simulink model "PSB3_0"  (R2021a)
settings: Solver=VariableStepAuto  StartTime=0.0  StopTime=3000  RelTol=1e-3
values from neighbouring files (symbols this model uses):
  n_channel = 1024    [PSB3_0_script.m]    (also in PSB_FPGAdesign8_script.m)
  parallel_factor = 4    [PSB3_0_script.m]    (also in PSB_FPGAdesign8_script.m)
libraries: xbsIndex_r4 x1051, xrbsSSR_Library x154, dspsrcs4 x26
(part 5 of 8)

== system PSB3_0/ov_detector_IFFT_im ==
  rst : Inport
  A : Inport  Port=2
  B : Inport  Port=3
  en : Inport  Port=4
  Constant17 : xbsIndex_r4/Constant  const=1  gui_display_data_type=Boolean  arith_type=Boolean  n_bits=16  bin_pt=14  preci_type=Single  exp_width=8  frac_width=24  explicit_period=on  period=1  equ=P=C  opselect=C  inp2=PCIN>>17  opr=+  inp1=P  carry=CIN  dbl_ovrd=off  block_type=constant
  Demux : Demux  Outputs=8
  Expression : xbsIndex_r4/Expression  expression=a1 | b1 | c1 | d1 | a2 | b2 | c2 | d2  align_bp=off  en=off  latency=1  precision=Full  arith_type=Unsigned  n_bits=1  bin_pt=0  dbl_ovrd=off  block_type=expr
  Register : xbsIndex_r4/Register  init=0  rst=on  en=on  dbl_ovrd=off  block_type=register
  Vector Absolute : xrbsSSR_Library/vector Absolute  precision=User Defined  arith_type="Signed  (2's comp)"  n_bits=20  bin_pt=15  quantization=Truncate  overflow=Saturate  en=off  sg_latency=1  dbl_ovrd=off  block_type=abs_ssr  sg_ssr_name=vect_absolute  sg_ssr=8  sg_ssr_prev=8
      settings: SourceProductName=Xilinx SSR Blockset
  Vector Absolute1 : xrbsSSR_Library/vector Absolute  precision=User Defined  arith_type="Signed  (2's comp)"  n_bits=20  bin_pt=15  quantization=Truncate  overflow=Saturate  en=off  sg_latency=1  dbl_ovrd=off  block_type=abs_ssr  sg_ssr_name=vect_absolute  sg_ssr=8  sg_ssr_prev=8
      settings: SourceProductName=Xilinx SSR Blockset
  Vector Register : xrbsSSR_Library/Vector Register  init=zeros(1,8)  en=on  rst=on  sg_ssr=8  sg_ssr_prev=8  sg_ssr_name=vect_reg  block_type=register_ssr  dbl_ovrd=off
      settings: SourceProductName=Xilinx SSR Blockset
  Vector Relational : xrbsSSR_Library/Vector Relational  mode=a>b  op_type=Bool  en=off  sg_latency=1  dbl_ovrd=off  has_advanced_contorl=0  block_type=relational_ssr  sg_ssr=8  sg_ssr_prev=8  sg_ssr_name=vect_relational
      settings: SourceProductName=Xilinx SSR Blockset
  ov : Outport
  wires:
  Demux/8 -> Expression/8
  Demux/7 -> Expression/7
  Demux/6 -> Expression/6
  Demux/5 -> Expression/5
  Demux/4 -> Expression/4
  Demux/3 -> Expression/3
  B/1 -> Vector Absolute1/1
  Vector Absolute1/1 -> Vector Relational/2
  Vector Absolute/1 -> Vector Relational/1
  Vector Register/1 -> Vector Absolute/1
  en/1 -> Vector Register/3
  A/1 -> Vector Register/1
  rst/1 -> Register/2, Vector Register/2
  Demux/1 -> Expression/1
  Vector Relational/1 -> Demux/1
  Register/1 -> ov/1
  Demux/2 -> Expression/2
  Constant17/1 -> Register/1
  Expression/1 -> Register/3

== system PSB3_0/ov_detector_IFFT_re ==
  rst : Inport
  A : Inport  Port=2
  B : Inport  Port=3
  en : Inport  Port=4
  Constant17 : xbsIndex_r4/Constant  const=1  gui_display_data_type=Boolean  arith_type=Boolean  n_bits=16  bin_pt=14  preci_type=Single  exp_width=8  frac_width=24  explicit_period=on  period=1  equ=P=C  opselect=C  inp2=PCIN>>17  opr=+  inp1=P  carry=CIN  dbl_ovrd=off  block_type=constant
  Demux : Demux  Outputs=8
  Expression : xbsIndex_r4/Expression  expression=a1 | b1 | c1 | d1 | a2 | b2 | c2 | d2  align_bp=off  en=off  latency=1  precision=Full  arith_type=Unsigned  n_bits=1  bin_pt=0  dbl_ovrd=off  block_type=expr
  Register : xbsIndex_r4/Register  init=0  rst=on  en=on  dbl_ovrd=off  block_type=register
  Vector Absolute : xrbsSSR_Library/vector Absolute  precision=User Defined  arith_type="Signed  (2's comp)"  n_bits=20  bin_pt=15  quantization=Truncate  overflow=Saturate  en=off  sg_latency=1  dbl_ovrd=off  block_type=abs_ssr  sg_ssr_name=vect_absolute  sg_ssr=8  sg_ssr_prev=8
      settings: SourceProductName=Xilinx SSR Blockset
  Vector Absolute1 : xrbsSSR_Library/vector Absolute  precision=User Defined  arith_type="Signed  (2's comp)"  n_bits=20  bin_pt=15  quantization=Truncate  overflow=Saturate  en=off  sg_latency=1  dbl_ovrd=off  block_type=abs_ssr  sg_ssr_name=vect_absolute  sg_ssr=8  sg_ssr_prev=8
      settings: SourceProductName=Xilinx SSR Blockset
  Vector Register : xrbsSSR_Library/Vector Register  init=zeros(1,8)  en=on  rst=on  sg_ssr=8  sg_ssr_prev=8  sg_ssr_name=vect_reg  block_type=register_ssr  dbl_ovrd=off
      settings: SourceProductName=Xilinx SSR Blockset
  Vector Relational : xrbsSSR_Library/Vector Relational  mode=a>b  op_type=Bool  en=off  sg_latency=1  dbl_ovrd=off  has_advanced_contorl=0  block_type=relational_ssr  sg_ssr=8  sg_ssr_prev=8  sg_ssr_name=vect_relational
      settings: SourceProductName=Xilinx SSR Blockset
  ov : Outport
  wires:
  Expression/1 -> Register/3
  Constant17/1 -> Register/1
  Demux/2 -> Expression/2
  Register/1 -> ov/1
  Vector Relational/1 -> Demux/1
  Demux/1 -> Expression/1
  rst/1 -> Vector Register/2, Register/2
  A/1 -> Vector Register/1
  en/1 -> Vector Register/3
  Vector Register/1 -> Vector Absolute/1
  Vector Absolute/1 -> Vector Relational/1
  Vector Absolute1/1 -> Vector Relational/2
  B/1 -> Vector Absolute1/1
  Demux/3 -> Expression/3
  Demux/4 -> Expression/4
  Demux/5 -> Expression/5
  Demux/6 -> Expression/6
  Demux/7 -> Expression/7
  Demux/8 -> Expression/8

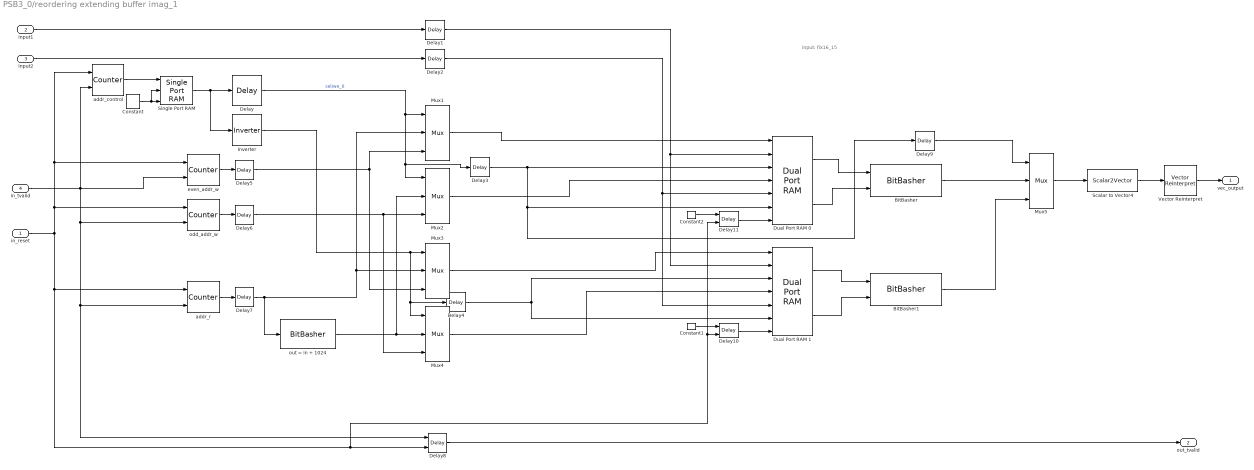
== system PSB3_0/reordering extending buffer imag_1 ==
  note: input: fix16_15
  in_reset : Inport
  input1 : Inport  Port=2
  input2 : Inport  Port=3
  in_tvalid : Inport  Port=4
  BitBasher : xbsIndex_r4/BitBasher  bitexpr=out = {8{b,a}}  display_expr=on  sr_1=out  arith_type1=Unsigned  bin_pt1=0  sr_2=2  arith_type2=Unsigned  bin_pt2=0  sr_3=3  arith_type3=Unsigned  bin_pt3=0  sr_4=4  arith_type4=Unsigned  bin_pt4=0  dbl_ovrd=off  block_type=bitbasher
  BitBasher1 : xbsIndex_r4/BitBasher  bitexpr=out = {8{b,a}}  display_expr=on  sr_1=out  arith_type1=Unsigned  bin_pt1=0  sr_2=2  arith_type2=Unsigned  bin_pt2=0  sr_3=3  arith_type3=Unsigned  bin_pt3=0  sr_4=4  arith_type4=Unsigned  bin_pt4=0  dbl_ovrd=off  block_type=bitbasher
  Constant : xbsIndex_r4/Constant  const=0  gui_display_data_type=Boolean  arith_type=Boolean  n_bits=16  bin_pt=14  preci_type=Single  exp_width=8  frac_width=24  explicit_period=on  period=1  equ=P=C  opselect=C  inp2=PCIN>>17  opr=+  inp1=P  carry=CIN  dbl_ovrd=off  block_type=constant
  Constant1 : xbsIndex_r4/Constant  const=1  gui_display_data_type=Boolean  arith_type=Boolean  n_bits=16  bin_pt=14  preci_type=Single  exp_width=8  frac_width=24  explicit_period=on  period=1  equ=P=C  opselect=C  inp2=PCIN>>17  opr=+  inp1=P  carry=CIN  dbl_ovrd=off  block_type=constant
  Constant2 : xbsIndex_r4/Constant  const=1  gui_display_data_type=Boolean  arith_type=Boolean  n_bits=16  bin_pt=14  preci_type=Single  exp_width=8  frac_width=24  explicit_period=on  period=1  equ=P=C  opselect=C  inp2=PCIN>>17  opr=+  inp1=P  carry=CIN  dbl_ovrd=off  block_type=constant
  Delay{,3..4,9} (4 alike) : xbsIndex_r4/Delay  rst=off  infoeditControl=Selection of Reset will increase slice count due to use of real FFs and instead of SRLs  en=off  latency=1  reg_retiming=off  dbl_ovrd=off  block_type=delay
  Delay1 : xbsIndex_r4/Delay  rst=off  infoeditControl=Selection of Reset will increase slice count due to use of real FFs and instead of SRLs  en=off  latency=3  reg_retiming=off  dbl_ovrd=off  block_type=delay
  Delay10 : xbsIndex_r4/Delay  rst=on  infoeditControl=Selection of Reset will increase slice count due to use of real FFs and instead of SRLs  en=off  latency=1000  reg_retiming=off  dbl_ovrd=off  block_type=delay
  Delay11 : xbsIndex_r4/Delay  rst=on  infoeditControl=Selection of Reset will increase slice count due to use of real FFs and instead of SRLs  en=off  latency=1000  reg_retiming=off  dbl_ovrd=off  block_type=delay
  Delay2 : xbsIndex_r4/Delay  rst=off  infoeditControl=Selection of Reset will increase slice count due to use of real FFs and instead of SRLs  en=off  latency=3  reg_retiming=off  dbl_ovrd=off  block_type=delay
  Delay5 : xbsIndex_r4/Delay  rst=off  infoeditControl=Selection of Reset will increase slice count due to use of real FFs and instead of SRLs  en=off  latency=2  reg_retiming=off  dbl_ovrd=off  block_type=delay
  Delay6 : xbsIndex_r4/Delay  rst=off  infoeditControl=Selection of Reset will increase slice count due to use of real FFs and instead of SRLs  en=off  latency=2  reg_retiming=off  dbl_ovrd=off  block_type=delay
  Delay7 : xbsIndex_r4/Delay  rst=off  infoeditControl=Selection of Reset will increase slice count due to use of real FFs and instead of SRLs  en=off  latency=2  reg_retiming=off  dbl_ovrd=off  block_type=delay
  Delay8 : xbsIndex_r4/Delay  rst=on  infoeditControl=Selection of Reset will increase slice count due to use of real FFs and instead of SRLs  en=off  latency=4+1024/parallel_factor+1 - 2  reg_retiming=off  dbl_ovrd=off  block_type=delay
  Dual Port RAM 0 : xbsIndex_r4/Dual Port RAM  depth=2048/parallel_factor  initVector=1  distributed_mem=Block RAM  init_a=0  init_b=0  rst_a=off  rst_b=off  en_a=off  en_b=on  latency=1  write_mode_A=Read Before Write  write_mode_B=Read Before Write  optimize=Area  dbl_ovrd=off  simulation_type=fast_sim  block_type=dpram
  Dual Port RAM 1 : xbsIndex_r4/Dual Port RAM  depth=2048/parallel_factor  initVector=1  distributed_mem=Block RAM  init_a=0  init_b=0  rst_a=off  rst_b=off  en_a=off  en_b=on  latency=1  write_mode_A=Read Before Write  write_mode_B=Read Before Write  optimize=Area  dbl_ovrd=off  simulation_type=fast_sim  block_type=dpram
  Inverter : xbsIndex_r4/Inverter  en=off  latency=1  dbl_ovrd=off  block_type=inv
  Mux{1..4} (4 alike) : xbsIndex_r4/Mux  inputs=2  en=off  latency=1  precision=Full  arith_type=Unsigned  n_bits=16  bin_pt=14  quantization=Truncate  overflow=Wrap  dbl_ovrd=off  block_type=mux
  Mux5 : xbsIndex_r4/Mux  inputs=2  en=off  latency=1  precision=User Defined  arith_type=Unsigned  n_bits=256  bin_pt=0  quantization=Truncate  overflow=Flag as error  dbl_ovrd=off  block_type=mux
  Scalar to Vector4 : xrbsSSR_Library/Scalar2Vector  Width=16  sg_ssr=16  sg_ssr_prev=16  sg_ssr_name=vect_Scalar2Vector  block_type=scalar2vector_ssr
      settings: SourceProductName=Xilinx SSR Blockset
  Single Port RAM : xbsIndex_r4/Single Port RAM  depth=2048/parallel_factor  initVector=[ones(1,1024/parallel_factor), zeros(1,1024/parallel_factor)]  distributed_mem=Block RAM  write_mode=Read Before Write  rst=off  init_reg=0  en=off  optimize_latency=off  latency=1  optimize=Area  dbl_ovrd=off  simulation_type=fast_sim  block_type=spram
  Vector Reinterpret : xrbsSSR_Library/Vector Reinterpret  sg_ssr=16  sg_ssr_prev=16  force_arith_type=on  arith_type="Signed  (2's comp)"  force_bin_pt=on  bin_pt=15  block_type=reinterpret_ssr
      settings: SourceProductName=Xilinx SSR Blockset  infoedit="The Vector Reinterpret block Changes vector input signal type without altering the binary representation. You can change the signal between signed and unsigned, and relocate the binary point.<br><br>Hardware notes: In hardware this block costs nothing.<br><br>Example:  Suppose the input is 6 bits wide, signed, with 2 fractional bits, and the output is forced to unsigned with 0 fractional bits.  Then an input of -2.0 (1110.00 in binary 2's complement) becomes an output of 56 (111000 in binary)."
  addr_control : xbsIndex_r4/Counter  cnt_type=Free Running  cnt_to=Inf  operation=Up  start_count=0  cnt_by_val=1  arith_type=Unsigned  n_bits=11-2  bin_pt=0  load_pin=off  rst=on  en=on  explicit_period=on  period=1  use_behavioral_HDL=off  implementation=Fabric  dbl_ovrd=off  block_type=counter
  addr_r : xbsIndex_r4/Counter  cnt_type=Free Running  cnt_to=Inf  operation=Up  start_count=0  cnt_by_val=1  arith_type=Unsigned  n_bits=10-2  bin_pt=0  load_pin=off  rst=on  en=on  explicit_period=on  period=1  use_behavioral_HDL=off  implementation=Fabric  dbl_ovrd=off  block_type=counter
  even_addr_w : xbsIndex_r4/Counter  cnt_type=Free Running  cnt_to=Inf  operation=Up  start_count=0  cnt_by_val=2  arith_type=Unsigned  n_bits=11-2  bin_pt=0  load_pin=off  rst=on  en=on  explicit_period=on  period=1  use_behavioral_HDL=off  implementation=Fabric  dbl_ovrd=off  block_type=counter
  odd_addr_w : xbsIndex_r4/Counter  cnt_type=Free Running  cnt_to=Inf  operation=Up  start_count=1  cnt_by_val=2  arith_type=Unsigned  n_bits=11-2  bin_pt=0  load_pin=off  rst=on  en=on  explicit_period=on  period=1  use_behavioral_HDL=off  implementation=Fabric  dbl_ovrd=off  block_type=counter
  out = in + 1024 : xbsIndex_r4/BitBasher  bitexpr=out={1'b1, in}  display_expr=on  sr_1=out  arith_type1=Unsigned  bin_pt1=0  sr_2=2  arith_type2=Unsigned  bin_pt2=0  sr_3=3  arith_type3=Unsigned  bin_pt3=0  sr_4=4  arith_type4=Unsigned  bin_pt4=0  dbl_ovrd=off  block_type=bitbasher
  vec_output : Outport
  out_tvalid : Outport  Port=2
  wires:
  in_reset/1 -> addr_control/1, even_addr_w/1, odd_addr_w/1, addr_r/1, Delay8/2, Delay10/2, Delay11/2
  Vector Reinterpret/1 -> vec_output/1
  Dual Port RAM 1/2 -> BitBasher1/2
  Dual Port RAM 0/2 -> BitBasher/2
  Delay10/1 -> Dual Port RAM 1/7
  Constant1/1 -> Delay10/1
  Delay11/1 -> Dual Port RAM 0/7
  Constant2/1 -> Delay11/1
  input2/1 -> Delay2/1
  input1/1 -> Delay1/1
  Scalar to Vector4/1 -> Vector Reinterpret/1
  BitBasher1/1 -> Mux5/3
  Delay4/1 -> Dual Port RAM 1/3, Dual Port RAM 1/6
  BitBasher/1 -> Mux5/2
  Delay5/1 -> Mux1/3, Mux3/3
  addr_control/1 -> Single Port RAM/1
  Delay2/1 -> Dual Port RAM 0/5, Dual Port RAM 1/5
  out = in + 1024/1 -> Mux4/2, Mux2/2
  Constant/1 -> Single Port RAM/3, Single Port RAM/2
  Inverter/1 -> Mux3/1, Mux4/1, Delay4/1
  Delay3/1 -> Delay9/1, Dual Port RAM 0/6, Dual Port RAM 0/3
  Single Port RAM/1 -> Delay/1, Inverter/1
  Mux3/1 -> Dual Port RAM 1/1
  Dual Port RAM 1/1 -> BitBasher1/1
  addr_r/1 -> Delay7/1
  Delay7/1 -> out = in + 1024/1, Mux3/2, Mux1/2
  Mux1/1 -> Dual Port RAM 0/1
  Mux5/1 -> Scalar to Vector4/1
  even_addr_w/1 -> Delay5/1
  Delay/1 -> Mux1/1, Mux2/1, Delay3/1  "sel/we_0"
  Delay8/1 -> out_tvalid/1
  Delay9/1 -> Mux5/1
  odd_addr_w/1 -> Delay6/1
  Mux4/1 -> Dual Port RAM 1/4
  in_tvalid/1 -> addr_control/2, even_addr_w/2, odd_addr_w/2, Delay8/1, addr_r/2
  Mux2/1 -> Dual Port RAM 0/4
  Delay1/1 -> Dual Port RAM 0/2, Dual Port RAM 1/2
  Dual Port RAM 0/1 -> BitBasher/1
  Delay6/1 -> Mux2/3, Mux4/3

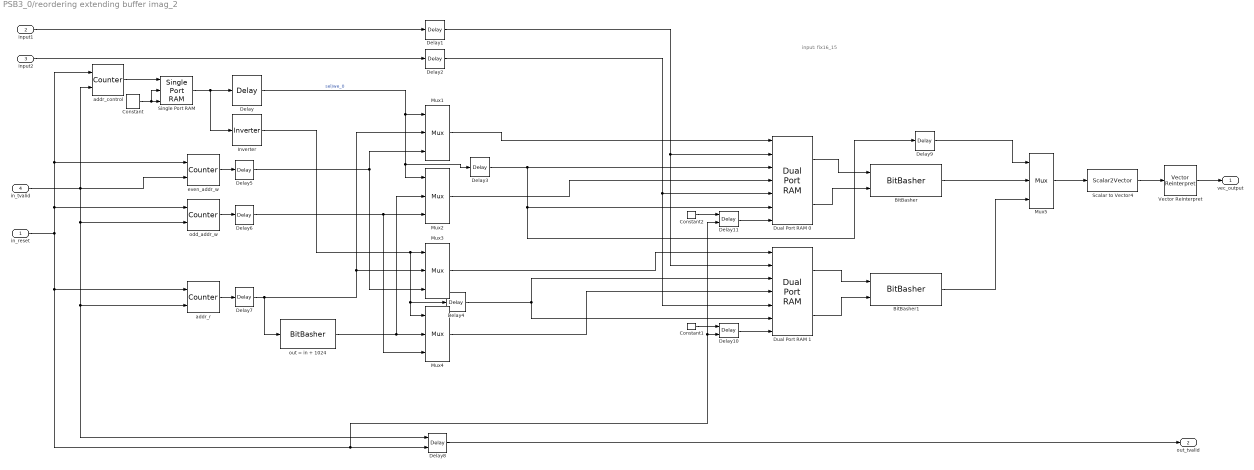
== system PSB3_0/reordering extending buffer imag_2 ==
  note: input: fix16_15
  in_reset : Inport
  input1 : Inport  Port=2
  input2 : Inport  Port=3
  in_tvalid : Inport  Port=4
  BitBasher : xbsIndex_r4/BitBasher  bitexpr=out = {8{b,a}}  display_expr=on  sr_1=out  arith_type1=Unsigned  bin_pt1=0  sr_2=2  arith_type2=Unsigned  bin_pt2=0  sr_3=3  arith_type3=Unsigned  bin_pt3=0  sr_4=4  arith_type4=Unsigned  bin_pt4=0  dbl_ovrd=off  block_type=bitbasher
  BitBasher1 : xbsIndex_r4/BitBasher  bitexpr=out = {8{b,a}}  display_expr=on  sr_1=out  arith_type1=Unsigned  bin_pt1=0  sr_2=2  arith_type2=Unsigned  bin_pt2=0  sr_3=3  arith_type3=Unsigned  bin_pt3=0  sr_4=4  arith_type4=Unsigned  bin_pt4=0  dbl_ovrd=off  block_type=bitbasher
  Constant : xbsIndex_r4/Constant  const=0  gui_display_data_type=Boolean  arith_type=Boolean  n_bits=16  bin_pt=14  preci_type=Single  exp_width=8  frac_width=24  explicit_period=on  period=1  equ=P=C  opselect=C  inp2=PCIN>>17  opr=+  inp1=P  carry=CIN  dbl_ovrd=off  block_type=constant
  Constant1 : xbsIndex_r4/Constant  const=1  gui_display_data_type=Boolean  arith_type=Boolean  n_bits=16  bin_pt=14  preci_type=Single  exp_width=8  frac_width=24  explicit_period=on  period=1  equ=P=C  opselect=C  inp2=PCIN>>17  opr=+  inp1=P  carry=CIN  dbl_ovrd=off  block_type=constant
  Constant2 : xbsIndex_r4/Constant  const=1  gui_display_data_type=Boolean  arith_type=Boolean  n_bits=16  bin_pt=14  preci_type=Single  exp_width=8  frac_width=24  explicit_period=on  period=1  equ=P=C  opselect=C  inp2=PCIN>>17  opr=+  inp1=P  carry=CIN  dbl_ovrd=off  block_type=constant
  Delay{,3..4,9} (4 alike) : xbsIndex_r4/Delay  rst=off  infoeditControl=Selection of Reset will increase slice count due to use of real FFs and instead of SRLs  en=off  latency=1  reg_retiming=off  dbl_ovrd=off  block_type=delay
  Delay1 : xbsIndex_r4/Delay  rst=off  infoeditControl=Selection of Reset will increase slice count due to use of real FFs and instead of SRLs  en=off  latency=3  reg_retiming=off  dbl_ovrd=off  block_type=delay
  Delay10 : xbsIndex_r4/Delay  rst=on  infoeditControl=Selection of Reset will increase slice count due to use of real FFs and instead of SRLs  en=off  latency=1000  reg_retiming=off  dbl_ovrd=off  block_type=delay
  Delay11 : xbsIndex_r4/Delay  rst=on  infoeditControl=Selection of Reset will increase slice count due to use of real FFs and instead of SRLs  en=off  latency=1000  reg_retiming=off  dbl_ovrd=off  block_type=delay
  Delay2 : xbsIndex_r4/Delay  rst=off  infoeditControl=Selection of Reset will increase slice count due to use of real FFs and instead of SRLs  en=off  latency=3  reg_retiming=off  dbl_ovrd=off  block_type=delay
  Delay5 : xbsIndex_r4/Delay  rst=off  infoeditControl=Selection of Reset will increase slice count due to use of real FFs and instead of SRLs  en=off  latency=2  reg_retiming=off  dbl_ovrd=off  block_type=delay
  Delay6 : xbsIndex_r4/Delay  rst=off  infoeditControl=Selection of Reset will increase slice count due to use of real FFs and instead of SRLs  en=off  latency=2  reg_retiming=off  dbl_ovrd=off  block_type=delay
  Delay7 : xbsIndex_r4/Delay  rst=off  infoeditControl=Selection of Reset will increase slice count due to use of real FFs and instead of SRLs  en=off  latency=2  reg_retiming=off  dbl_ovrd=off  block_type=delay
  Delay8 : xbsIndex_r4/Delay  rst=on  infoeditControl=Selection of Reset will increase slice count due to use of real FFs and instead of SRLs  en=off  latency=4+1024/parallel_factor+1 - 2  reg_retiming=off  dbl_ovrd=off  block_type=delay
  Dual Port RAM 0 : xbsIndex_r4/Dual Port RAM  depth=2048/parallel_factor  initVector=1  distributed_mem=Block RAM  init_a=0  init_b=0  rst_a=off  rst_b=off  en_a=off  en_b=on  latency=1  write_mode_A=Read Before Write  write_mode_B=Read Before Write  optimize=Area  dbl_ovrd=off  simulation_type=fast_sim  block_type=dpram
  Dual Port RAM 1 : xbsIndex_r4/Dual Port RAM  depth=2048/parallel_factor  initVector=1  distributed_mem=Block RAM  init_a=0  init_b=0  rst_a=off  rst_b=off  en_a=off  en_b=on  latency=1  write_mode_A=Read Before Write  write_mode_B=Read Before Write  optimize=Area  dbl_ovrd=off  simulation_type=fast_sim  block_type=dpram
  Inverter : xbsIndex_r4/Inverter  en=off  latency=1  dbl_ovrd=off  block_type=inv
  Mux{1..4} (4 alike) : xbsIndex_r4/Mux  inputs=2  en=off  latency=1  precision=Full  arith_type=Unsigned  n_bits=16  bin_pt=14  quantization=Truncate  overflow=Wrap  dbl_ovrd=off  block_type=mux
  Mux5 : xbsIndex_r4/Mux  inputs=2  en=off  latency=1  precision=User Defined  arith_type=Unsigned  n_bits=256  bin_pt=0  quantization=Truncate  overflow=Flag as error  dbl_ovrd=off  block_type=mux
  Scalar to Vector4 : xrbsSSR_Library/Scalar2Vector  Width=16  sg_ssr=16  sg_ssr_prev=16  sg_ssr_name=vect_Scalar2Vector  block_type=scalar2vector_ssr
      settings: SourceProductName=Xilinx SSR Blockset
  Single Port RAM : xbsIndex_r4/Single Port RAM  depth=2048/parallel_factor  initVector=[ones(1,1024/parallel_factor), zeros(1,1024/parallel_factor)]  distributed_mem=Block RAM  write_mode=Read Before Write  rst=off  init_reg=0  en=off  optimize_latency=off  latency=1  optimize=Area  dbl_ovrd=off  simulation_type=fast_sim  block_type=spram
  Vector Reinterpret : xrbsSSR_Library/Vector Reinterpret  sg_ssr=16  sg_ssr_prev=16  force_arith_type=on  arith_type="Signed  (2's comp)"  force_bin_pt=on  bin_pt=15  block_type=reinterpret_ssr
      settings: SourceProductName=Xilinx SSR Blockset  infoedit="The Vector Reinterpret block Changes vector input signal type without altering the binary representation. You can change the signal between signed and unsigned, and relocate the binary point.<br><br>Hardware notes: In hardware this block costs nothing.<br><br>Example:  Suppose the input is 6 bits wide, signed, with 2 fractional bits, and the output is forced to unsigned with 0 fractional bits.  Then an input of -2.0 (1110.00 in binary 2's complement) becomes an output of 56 (111000 in binary)."
  addr_control : xbsIndex_r4/Counter  cnt_type=Free Running  cnt_to=Inf  operation=Up  start_count=0  cnt_by_val=1  arith_type=Unsigned  n_bits=11-2  bin_pt=0  load_pin=off  rst=on  en=on  explicit_period=on  period=1  use_behavioral_HDL=off  implementation=Fabric  dbl_ovrd=off  block_type=counter
  addr_r : xbsIndex_r4/Counter  cnt_type=Free Running  cnt_to=Inf  operation=Up  start_count=0  cnt_by_val=1  arith_type=Unsigned  n_bits=10-2  bin_pt=0  load_pin=off  rst=on  en=on  explicit_period=on  period=1  use_behavioral_HDL=off  implementation=Fabric  dbl_ovrd=off  block_type=counter
  even_addr_w : xbsIndex_r4/Counter  cnt_type=Free Running  cnt_to=Inf  operation=Up  start_count=0  cnt_by_val=2  arith_type=Unsigned  n_bits=11-2  bin_pt=0  load_pin=off  rst=on  en=on  explicit_period=on  period=1  use_behavioral_HDL=off  implementation=Fabric  dbl_ovrd=off  block_type=counter
  odd_addr_w : xbsIndex_r4/Counter  cnt_type=Free Running  cnt_to=Inf  operation=Up  start_count=1  cnt_by_val=2  arith_type=Unsigned  n_bits=11-2  bin_pt=0  load_pin=off  rst=on  en=on  explicit_period=on  period=1  use_behavioral_HDL=off  implementation=Fabric  dbl_ovrd=off  block_type=counter
  out = in + 1024 : xbsIndex_r4/BitBasher  bitexpr=out={1'b1, in}  display_expr=on  sr_1=out  arith_type1=Unsigned  bin_pt1=0  sr_2=2  arith_type2=Unsigned  bin_pt2=0  sr_3=3  arith_type3=Unsigned  bin_pt3=0  sr_4=4  arith_type4=Unsigned  bin_pt4=0  dbl_ovrd=off  block_type=bitbasher
  vec_output : Outport
  out_tvalid : Outport  Port=2
  wires:
  in_reset/1 -> addr_control/1, even_addr_w/1, odd_addr_w/1, addr_r/1, Delay8/2, Delay10/2, Delay11/2
  Vector Reinterpret/1 -> vec_output/1
  Dual Port RAM 1/2 -> BitBasher1/2
  Dual Port RAM 0/2 -> BitBasher/2
  Delay10/1 -> Dual Port RAM 1/7
  Constant1/1 -> Delay10/1
  Delay11/1 -> Dual Port RAM 0/7
  Constant2/1 -> Delay11/1
  input2/1 -> Delay2/1
  input1/1 -> Delay1/1
  Scalar to Vector4/1 -> Vector Reinterpret/1
  BitBasher1/1 -> Mux5/3
  Delay4/1 -> Dual Port RAM 1/3, Dual Port RAM 1/6
  BitBasher/1 -> Mux5/2
  Delay5/1 -> Mux1/3, Mux3/3
  addr_control/1 -> Single Port RAM/1
  Delay2/1 -> Dual Port RAM 0/5, Dual Port RAM 1/5
  out = in + 1024/1 -> Mux4/2, Mux2/2
  Constant/1 -> Single Port RAM/3, Single Port RAM/2
  Inverter/1 -> Mux3/1, Mux4/1, Delay4/1
  Delay3/1 -> Delay9/1, Dual Port RAM 0/6, Dual Port RAM 0/3
  Single Port RAM/1 -> Delay/1, Inverter/1
  Mux3/1 -> Dual Port RAM 1/1
  Dual Port RAM 1/1 -> BitBasher1/1
  addr_r/1 -> Delay7/1
  Delay7/1 -> out = in + 1024/1, Mux3/2, Mux1/2
  Mux1/1 -> Dual Port RAM 0/1
  Mux5/1 -> Scalar to Vector4/1
  even_addr_w/1 -> Delay5/1
  Delay/1 -> Mux1/1, Mux2/1, Delay3/1  "sel/we_0"
  Delay8/1 -> out_tvalid/1
  Delay9/1 -> Mux5/1
  odd_addr_w/1 -> Delay6/1
  Mux4/1 -> Dual Port RAM 1/4
  in_tvalid/1 -> addr_control/2, even_addr_w/2, odd_addr_w/2, Delay8/1, addr_r/2
  Mux2/1 -> Dual Port RAM 0/4
  Delay1/1 -> Dual Port RAM 0/2, Dual Port RAM 1/2
  Dual Port RAM 0/1 -> BitBasher/1
  Delay6/1 -> Mux2/3, Mux4/3

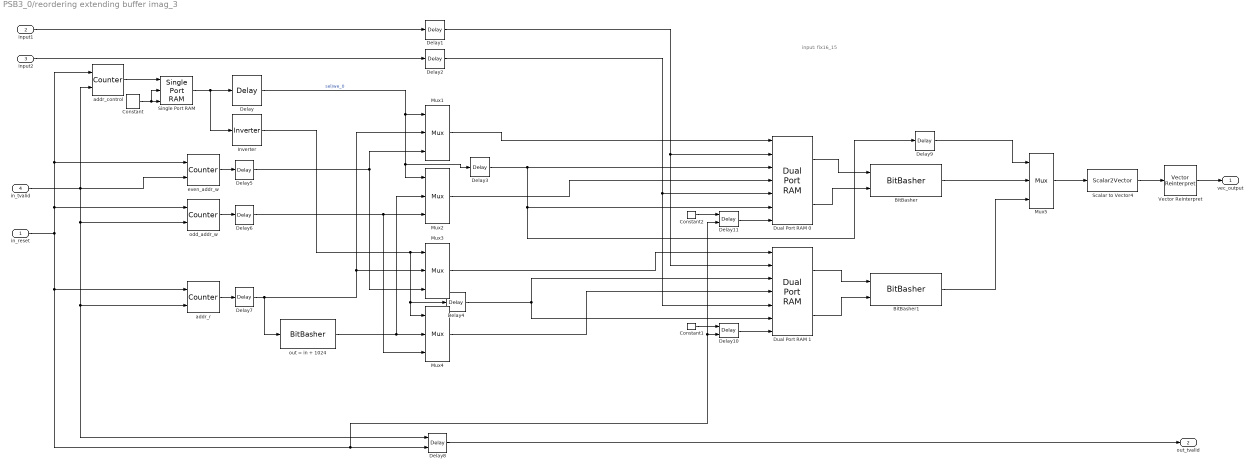
== system PSB3_0/reordering extending buffer imag_3 ==
  note: input: fix16_15
  in_reset : Inport
  input1 : Inport  Port=2
  input2 : Inport  Port=3
  in_tvalid : Inport  Port=4
  BitBasher : xbsIndex_r4/BitBasher  bitexpr=out = {8{b,a}}  display_expr=on  sr_1=out  arith_type1=Unsigned  bin_pt1=0  sr_2=2  arith_type2=Unsigned  bin_pt2=0  sr_3=3  arith_type3=Unsigned  bin_pt3=0  sr_4=4  arith_type4=Unsigned  bin_pt4=0  dbl_ovrd=off  block_type=bitbasher
  BitBasher1 : xbsIndex_r4/BitBasher  bitexpr=out = {8{b,a}}  display_expr=on  sr_1=out  arith_type1=Unsigned  bin_pt1=0  sr_2=2  arith_type2=Unsigned  bin_pt2=0  sr_3=3  arith_type3=Unsigned  bin_pt3=0  sr_4=4  arith_type4=Unsigned  bin_pt4=0  dbl_ovrd=off  block_type=bitbasher
  Constant : xbsIndex_r4/Constant  const=0  gui_display_data_type=Boolean  arith_type=Boolean  n_bits=16  bin_pt=14  preci_type=Single  exp_width=8  frac_width=24  explicit_period=on  period=1  equ=P=C  opselect=C  inp2=PCIN>>17  opr=+  inp1=P  carry=CIN  dbl_ovrd=off  block_type=constant
  Constant1 : xbsIndex_r4/Constant  const=1  gui_display_data_type=Boolean  arith_type=Boolean  n_bits=16  bin_pt=14  preci_type=Single  exp_width=8  frac_width=24  explicit_period=on  period=1  equ=P=C  opselect=C  inp2=PCIN>>17  opr=+  inp1=P  carry=CIN  dbl_ovrd=off  block_type=constant
  Constant2 : xbsIndex_r4/Constant  const=1  gui_display_data_type=Boolean  arith_type=Boolean  n_bits=16  bin_pt=14  preci_type=Single  exp_width=8  frac_width=24  explicit_period=on  period=1  equ=P=C  opselect=C  inp2=PCIN>>17  opr=+  inp1=P  carry=CIN  dbl_ovrd=off  block_type=constant
  Delay{,3..4,9} (4 alike) : xbsIndex_r4/Delay  rst=off  infoeditControl=Selection of Reset will increase slice count due to use of real FFs and instead of SRLs  en=off  latency=1  reg_retiming=off  dbl_ovrd=off  block_type=delay
  Delay1 : xbsIndex_r4/Delay  rst=off  infoeditControl=Selection of Reset will increase slice count due to use of real FFs and instead of SRLs  en=off  latency=3  reg_retiming=off  dbl_ovrd=off  block_type=delay
  Delay10 : xbsIndex_r4/Delay  rst=on  infoeditControl=Selection of Reset will increase slice count due to use of real FFs and instead of SRLs  en=off  latency=1000  reg_retiming=off  dbl_ovrd=off  block_type=delay
  Delay11 : xbsIndex_r4/Delay  rst=on  infoeditControl=Selection of Reset will increase slice count due to use of real FFs and instead of SRLs  en=off  latency=1000  reg_retiming=off  dbl_ovrd=off  block_type=delay
  Delay2 : xbsIndex_r4/Delay  rst=off  infoeditControl=Selection of Reset will increase slice count due to use of real FFs and instead of SRLs  en=off  latency=3  reg_retiming=off  dbl_ovrd=off  block_type=delay
  Delay5 : xbsIndex_r4/Delay  rst=off  infoeditControl=Selection of Reset will increase slice count due to use of real FFs and instead of SRLs  en=off  latency=2  reg_retiming=off  dbl_ovrd=off  block_type=delay
  Delay6 : xbsIndex_r4/Delay  rst=off  infoeditControl=Selection of Reset will increase slice count due to use of real FFs and instead of SRLs  en=off  latency=2  reg_retiming=off  dbl_ovrd=off  block_type=delay
  Delay7 : xbsIndex_r4/Delay  rst=off  infoeditControl=Selection of Reset will increase slice count due to use of real FFs and instead of SRLs  en=off  latency=2  reg_retiming=off  dbl_ovrd=off  block_type=delay
  Delay8 : xbsIndex_r4/Delay  rst=on  infoeditControl=Selection of Reset will increase slice count due to use of real FFs and instead of SRLs  en=off  latency=4+1024/parallel_factor+1 - 2  reg_retiming=off  dbl_ovrd=off  block_type=delay
  Dual Port RAM 0 : xbsIndex_r4/Dual Port RAM  depth=2048/parallel_factor  initVector=1  distributed_mem=Block RAM  init_a=0  init_b=0  rst_a=off  rst_b=off  en_a=off  en_b=on  latency=1  write_mode_A=Read Before Write  write_mode_B=Read Before Write  optimize=Area  dbl_ovrd=off  simulation_type=fast_sim  block_type=dpram
  Dual Port RAM 1 : xbsIndex_r4/Dual Port RAM  depth=2048/parallel_factor  initVector=1  distributed_mem=Block RAM  init_a=0  init_b=0  rst_a=off  rst_b=off  en_a=off  en_b=on  latency=1  write_mode_A=Read Before Write  write_mode_B=Read Before Write  optimize=Area  dbl_ovrd=off  simulation_type=fast_sim  block_type=dpram
  Inverter : xbsIndex_r4/Inverter  en=off  latency=1  dbl_ovrd=off  block_type=inv
  Mux{1..4} (4 alike) : xbsIndex_r4/Mux  inputs=2  en=off  latency=1  precision=Full  arith_type=Unsigned  n_bits=16  bin_pt=14  quantization=Truncate  overflow=Wrap  dbl_ovrd=off  block_type=mux
  Mux5 : xbsIndex_r4/Mux  inputs=2  en=off  latency=1  precision=User Defined  arith_type=Unsigned  n_bits=256  bin_pt=0  quantization=Truncate  overflow=Flag as error  dbl_ovrd=off  block_type=mux
  Scalar to Vector4 : xrbsSSR_Library/Scalar2Vector  Width=16  sg_ssr=16  sg_ssr_prev=16  sg_ssr_name=vect_Scalar2Vector  block_type=scalar2vector_ssr
      settings: SourceProductName=Xilinx SSR Blockset
  Single Port RAM : xbsIndex_r4/Single Port RAM  depth=2048/parallel_factor  initVector=[ones(1,1024/parallel_factor), zeros(1,1024/parallel_factor)]  distributed_mem=Block RAM  write_mode=Read Before Write  rst=off  init_reg=0  en=off  optimize_latency=off  latency=1  optimize=Area  dbl_ovrd=off  simulation_type=fast_sim  block_type=spram
  Vector Reinterpret : xrbsSSR_Library/Vector Reinterpret  sg_ssr=16  sg_ssr_prev=16  force_arith_type=on  arith_type="Signed  (2's comp)"  force_bin_pt=on  bin_pt=15  block_type=reinterpret_ssr
      settings: SourceProductName=Xilinx SSR Blockset  infoedit="The Vector Reinterpret block Changes vector input signal type without altering the binary representation. You can change the signal between signed and unsigned, and relocate the binary point.<br><br>Hardware notes: In hardware this block costs nothing.<br><br>Example:  Suppose the input is 6 bits wide, signed, with 2 fractional bits, and the output is forced to unsigned with 0 fractional bits.  Then an input of -2.0 (1110.00 in binary 2's complement) becomes an output of 56 (111000 in binary)."
  addr_control : xbsIndex_r4/Counter  cnt_type=Free Running  cnt_to=Inf  operation=Up  start_count=0  cnt_by_val=1  arith_type=Unsigned  n_bits=11-2  bin_pt=0  load_pin=off  rst=on  en=on  explicit_period=on  period=1  use_behavioral_HDL=off  implementation=Fabric  dbl_ovrd=off  block_type=counter
  addr_r : xbsIndex_r4/Counter  cnt_type=Free Running  cnt_to=Inf  operation=Up  start_count=0  cnt_by_val=1  arith_type=Unsigned  n_bits=10-2  bin_pt=0  load_pin=off  rst=on  en=on  explicit_period=on  period=1  use_behavioral_HDL=off  implementation=Fabric  dbl_ovrd=off  block_type=counter
  even_addr_w : xbsIndex_r4/Counter  cnt_type=Free Running  cnt_to=Inf  operation=Up  start_count=0  cnt_by_val=2  arith_type=Unsigned  n_bits=11-2  bin_pt=0  load_pin=off  rst=on  en=on  explicit_period=on  period=1  use_behavioral_HDL=off  implementation=Fabric  dbl_ovrd=off  block_type=counter
  odd_addr_w : xbsIndex_r4/Counter  cnt_type=Free Running  cnt_to=Inf  operation=Up  start_count=1  cnt_by_val=2  arith_type=Unsigned  n_bits=11-2  bin_pt=0  load_pin=off  rst=on  en=on  explicit_period=on  period=1  use_behavioral_HDL=off  implementation=Fabric  dbl_ovrd=off  block_type=counter
  out = in + 1024 : xbsIndex_r4/BitBasher  bitexpr=out={1'b1, in}  display_expr=on  sr_1=out  arith_type1=Unsigned  bin_pt1=0  sr_2=2  arith_type2=Unsigned  bin_pt2=0  sr_3=3  arith_type3=Unsigned  bin_pt3=0  sr_4=4  arith_type4=Unsigned  bin_pt4=0  dbl_ovrd=off  block_type=bitbasher
  vec_output : Outport
  out_tvalid : Outport  Port=2
  wires:
  in_reset/1 -> addr_control/1, even_addr_w/1, odd_addr_w/1, addr_r/1, Delay8/2, Delay10/2, Delay11/2
  Vector Reinterpret/1 -> vec_output/1
  Dual Port RAM 1/2 -> BitBasher1/2
  Dual Port RAM 0/2 -> BitBasher/2
  Delay10/1 -> Dual Port RAM 1/7
  Constant1/1 -> Delay10/1
  Delay11/1 -> Dual Port RAM 0/7
  Constant2/1 -> Delay11/1
  input2/1 -> Delay2/1
  input1/1 -> Delay1/1
  Scalar to Vector4/1 -> Vector Reinterpret/1
  BitBasher1/1 -> Mux5/3
  Delay4/1 -> Dual Port RAM 1/3, Dual Port RAM 1/6
  BitBasher/1 -> Mux5/2
  Delay5/1 -> Mux1/3, Mux3/3
  addr_control/1 -> Single Port RAM/1
  Delay2/1 -> Dual Port RAM 0/5, Dual Port RAM 1/5
  out = in + 1024/1 -> Mux4/2, Mux2/2
  Constant/1 -> Single Port RAM/3, Single Port RAM/2
  Inverter/1 -> Mux3/1, Mux4/1, Delay4/1
  Delay3/1 -> Delay9/1, Dual Port RAM 0/6, Dual Port RAM 0/3
  Single Port RAM/1 -> Delay/1, Inverter/1
  Mux3/1 -> Dual Port RAM 1/1
  Dual Port RAM 1/1 -> BitBasher1/1
  addr_r/1 -> Delay7/1
  Delay7/1 -> out = in + 1024/1, Mux3/2, Mux1/2
  Mux1/1 -> Dual Port RAM 0/1
  Mux5/1 -> Scalar to Vector4/1
  even_addr_w/1 -> Delay5/1
  Delay/1 -> Mux1/1, Mux2/1, Delay3/1  "sel/we_0"
  Delay8/1 -> out_tvalid/1
  Delay9/1 -> Mux5/1
  odd_addr_w/1 -> Delay6/1
  Mux4/1 -> Dual Port RAM 1/4
  in_tvalid/1 -> addr_control/2, even_addr_w/2, odd_addr_w/2, Delay8/1, addr_r/2
  Mux2/1 -> Dual Port RAM 0/4
  Delay1/1 -> Dual Port RAM 0/2, Dual Port RAM 1/2
  Dual Port RAM 0/1 -> BitBasher/1
  Delay6/1 -> Mux2/3, Mux4/3

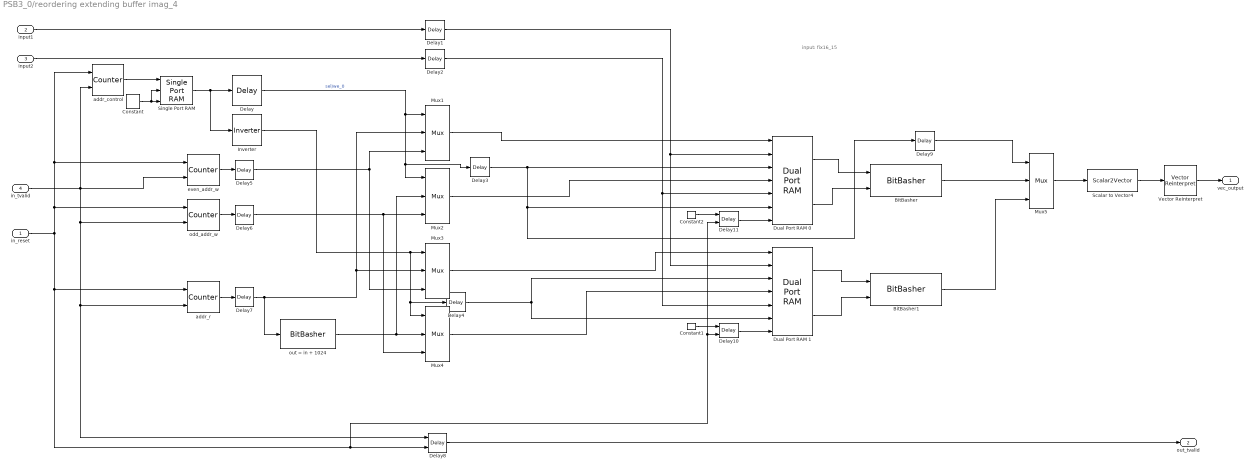
== system PSB3_0/reordering extending buffer imag_4 ==
  note: input: fix16_15
  in_reset : Inport
  input1 : Inport  Port=2
  input2 : Inport  Port=3
  in_tvalid : Inport  Port=4
  BitBasher : xbsIndex_r4/BitBasher  bitexpr=out = {8{b,a}}  display_expr=on  sr_1=out  arith_type1=Unsigned  bin_pt1=0  sr_2=2  arith_type2=Unsigned  bin_pt2=0  sr_3=3  arith_type3=Unsigned  bin_pt3=0  sr_4=4  arith_type4=Unsigned  bin_pt4=0  dbl_ovrd=off  block_type=bitbasher
  BitBasher1 : xbsIndex_r4/BitBasher  bitexpr=out = {8{b,a}}  display_expr=on  sr_1=out  arith_type1=Unsigned  bin_pt1=0  sr_2=2  arith_type2=Unsigned  bin_pt2=0  sr_3=3  arith_type3=Unsigned  bin_pt3=0  sr_4=4  arith_type4=Unsigned  bin_pt4=0  dbl_ovrd=off  block_type=bitbasher
  Constant : xbsIndex_r4/Constant  const=0  gui_display_data_type=Boolean  arith_type=Boolean  n_bits=16  bin_pt=14  preci_type=Single  exp_width=8  frac_width=24  explicit_period=on  period=1  equ=P=C  opselect=C  inp2=PCIN>>17  opr=+  inp1=P  carry=CIN  dbl_ovrd=off  block_type=constant
  Constant1 : xbsIndex_r4/Constant  const=1  gui_display_data_type=Boolean  arith_type=Boolean  n_bits=16  bin_pt=14  preci_type=Single  exp_width=8  frac_width=24  explicit_period=on  period=1  equ=P=C  opselect=C  inp2=PCIN>>17  opr=+  inp1=P  carry=CIN  dbl_ovrd=off  block_type=constant
  Constant2 : xbsIndex_r4/Constant  const=1  gui_display_data_type=Boolean  arith_type=Boolean  n_bits=16  bin_pt=14  preci_type=Single  exp_width=8  frac_width=24  explicit_period=on  period=1  equ=P=C  opselect=C  inp2=PCIN>>17  opr=+  inp1=P  carry=CIN  dbl_ovrd=off  block_type=constant
  Delay{,3..4,9} (4 alike) : xbsIndex_r4/Delay  rst=off  infoeditControl=Selection of Reset will increase slice count due to use of real FFs and instead of SRLs  en=off  latency=1  reg_retiming=off  dbl_ovrd=off  block_type=delay
  Delay1 : xbsIndex_r4/Delay  rst=off  infoeditControl=Selection of Reset will increase slice count due to use of real FFs and instead of SRLs  en=off  latency=3  reg_retiming=off  dbl_ovrd=off  block_type=delay
  Delay10 : xbsIndex_r4/Delay  rst=on  infoeditControl=Selection of Reset will increase slice count due to use of real FFs and instead of SRLs  en=off  latency=1000  reg_retiming=off  dbl_ovrd=off  block_type=delay
  Delay11 : xbsIndex_r4/Delay  rst=on  infoeditControl=Selection of Reset will increase slice count due to use of real FFs and instead of SRLs  en=off  latency=1000  reg_retiming=off  dbl_ovrd=off  block_type=delay
  Delay2 : xbsIndex_r4/Delay  rst=off  infoeditControl=Selection of Reset will increase slice count due to use of real FFs and instead of SRLs  en=off  latency=3  reg_retiming=off  dbl_ovrd=off  block_type=delay
  Delay5 : xbsIndex_r4/Delay  rst=off  infoeditControl=Selection of Reset will increase slice count due to use of real FFs and instead of SRLs  en=off  latency=2  reg_retiming=off  dbl_ovrd=off  block_type=delay
  Delay6 : xbsIndex_r4/Delay  rst=off  infoeditControl=Selection of Reset will increase slice count due to use of real FFs and instead of SRLs  en=off  latency=2  reg_retiming=off  dbl_ovrd=off  block_type=delay
  Delay7 : xbsIndex_r4/Delay  rst=off  infoeditControl=Selection of Reset will increase slice count due to use of real FFs and instead of SRLs  en=off  latency=2  reg_retiming=off  dbl_ovrd=off  block_type=delay
  Delay8 : xbsIndex_r4/Delay  rst=on  infoeditControl=Selection of Reset will increase slice count due to use of real FFs and instead of SRLs  en=off  latency=4+1024/parallel_factor+1 - 2  reg_retiming=off  dbl_ovrd=off  block_type=delay
  Dual Port RAM 0 : xbsIndex_r4/Dual Port RAM  depth=2048/parallel_factor  initVector=1  distributed_mem=Block RAM  init_a=0  init_b=0  rst_a=off  rst_b=off  en_a=off  en_b=on  latency=1  write_mode_A=Read Before Write  write_mode_B=Read Before Write  optimize=Area  dbl_ovrd=off  simulation_type=fast_sim  block_type=dpram
  Dual Port RAM 1 : xbsIndex_r4/Dual Port RAM  depth=2048/parallel_factor  initVector=1  distributed_mem=Block RAM  init_a=0  init_b=0  rst_a=off  rst_b=off  en_a=off  en_b=on  latency=1  write_mode_A=Read Before Write  write_mode_B=Read Before Write  optimize=Area  dbl_ovrd=off  simulation_type=fast_sim  block_type=dpram
  Inverter : xbsIndex_r4/Inverter  en=off  latency=1  dbl_ovrd=off  block_type=inv
  Mux{1..4} (4 alike) : xbsIndex_r4/Mux  inputs=2  en=off  latency=1  precision=Full  arith_type=Unsigned  n_bits=16  bin_pt=14  quantization=Truncate  overflow=Wrap  dbl_ovrd=off  block_type=mux
  Mux5 : xbsIndex_r4/Mux  inputs=2  en=off  latency=1  precision=User Defined  arith_type=Unsigned  n_bits=256  bin_pt=0  quantization=Truncate  overflow=Flag as error  dbl_ovrd=off  block_type=mux
  Scalar to Vector4 : xrbsSSR_Library/Scalar2Vector  Width=16  sg_ssr=16  sg_ssr_prev=16  sg_ssr_name=vect_Scalar2Vector  block_type=scalar2vector_ssr
      settings: SourceProductName=Xilinx SSR Blockset
  Single Port RAM : xbsIndex_r4/Single Port RAM  depth=2048/parallel_factor  initVector=[ones(1,1024/parallel_factor), zeros(1,1024/parallel_factor)]  distributed_mem=Block RAM  write_mode=Read Before Write  rst=off  init_reg=0  en=off  optimize_latency=off  latency=1  optimize=Area  dbl_ovrd=off  simulation_type=fast_sim  block_type=spram
  Vector Reinterpret : xrbsSSR_Library/Vector Reinterpret  sg_ssr=16  sg_ssr_prev=16  force_arith_type=on  arith_type="Signed  (2's comp)"  force_bin_pt=on  bin_pt=15  block_type=reinterpret_ssr
      settings: SourceProductName=Xilinx SSR Blockset  infoedit="The Vector Reinterpret block Changes vector input signal type without altering the binary representation. You can change the signal between signed and unsigned, and relocate the binary point.<br><br>Hardware notes: In hardware this block costs nothing.<br><br>Example:  Suppose the input is 6 bits wide, signed, with 2 fractional bits, and the output is forced to unsigned with 0 fractional bits.  Then an input of -2.0 (1110.00 in binary 2's complement) becomes an output of 56 (111000 in binary)."
  addr_control : xbsIndex_r4/Counter  cnt_type=Free Running  cnt_to=Inf  operation=Up  start_count=0  cnt_by_val=1  arith_type=Unsigned  n_bits=11-2  bin_pt=0  load_pin=off  rst=on  en=on  explicit_period=on  period=1  use_behavioral_HDL=off  implementation=Fabric  dbl_ovrd=off  block_type=counter
  addr_r : xbsIndex_r4/Counter  cnt_type=Free Running  cnt_to=Inf  operation=Up  start_count=0  cnt_by_val=1  arith_type=Unsigned  n_bits=10-2  bin_pt=0  load_pin=off  rst=on  en=on  explicit_period=on  period=1  use_behavioral_HDL=off  implementation=Fabric  dbl_ovrd=off  block_type=counter
  even_addr_w : xbsIndex_r4/Counter  cnt_type=Free Running  cnt_to=Inf  operation=Up  start_count=0  cnt_by_val=2  arith_type=Unsigned  n_bits=11-2  bin_pt=0  load_pin=off  rst=on  en=on  explicit_period=on  period=1  use_behavioral_HDL=off  implementation=Fabric  dbl_ovrd=off  block_type=counter
  odd_addr_w : xbsIndex_r4/Counter  cnt_type=Free Running  cnt_to=Inf  operation=Up  start_count=1  cnt_by_val=2  arith_type=Unsigned  n_bits=11-2  bin_pt=0  load_pin=off  rst=on  en=on  explicit_period=on  period=1  use_behavioral_HDL=off  implementation=Fabric  dbl_ovrd=off  block_type=counter
  out = in + 1024 : xbsIndex_r4/BitBasher  bitexpr=out={1'b1, in}  display_expr=on  sr_1=out  arith_type1=Unsigned  bin_pt1=0  sr_2=2  arith_type2=Unsigned  bin_pt2=0  sr_3=3  arith_type3=Unsigned  bin_pt3=0  sr_4=4  arith_type4=Unsigned  bin_pt4=0  dbl_ovrd=off  block_type=bitbasher
  vec_output : Outport
  out_tvalid : Outport  Port=2
  wires:
  in_reset/1 -> addr_control/1, even_addr_w/1, odd_addr_w/1, addr_r/1, Delay8/2, Delay10/2, Delay11/2
  Vector Reinterpret/1 -> vec_output/1
  Dual Port RAM 1/2 -> BitBasher1/2
  Dual Port RAM 0/2 -> BitBasher/2
  Delay10/1 -> Dual Port RAM 1/7
  Constant1/1 -> Delay10/1
  Delay11/1 -> Dual Port RAM 0/7
  Constant2/1 -> Delay11/1
  input2/1 -> Delay2/1
  input1/1 -> Delay1/1
  Scalar to Vector4/1 -> Vector Reinterpret/1
  BitBasher1/1 -> Mux5/3
  Delay4/1 -> Dual Port RAM 1/3, Dual Port RAM 1/6
  BitBasher/1 -> Mux5/2
  Delay5/1 -> Mux1/3, Mux3/3
  addr_control/1 -> Single Port RAM/1
  Delay2/1 -> Dual Port RAM 0/5, Dual Port RAM 1/5
  out = in + 1024/1 -> Mux4/2, Mux2/2
  Constant/1 -> Single Port RAM/3, Single Port RAM/2
  Inverter/1 -> Mux3/1, Mux4/1, Delay4/1
  Delay3/1 -> Delay9/1, Dual Port RAM 0/6, Dual Port RAM 0/3
  Single Port RAM/1 -> Delay/1, Inverter/1
  Mux3/1 -> Dual Port RAM 1/1
  Dual Port RAM 1/1 -> BitBasher1/1
  addr_r/1 -> Delay7/1
  Delay7/1 -> out = in + 1024/1, Mux3/2, Mux1/2
  Mux1/1 -> Dual Port RAM 0/1
  Mux5/1 -> Scalar to Vector4/1
  even_addr_w/1 -> Delay5/1
  Delay/1 -> Mux1/1, Mux2/1, Delay3/1  "sel/we_0"
  Delay8/1 -> out_tvalid/1
  Delay9/1 -> Mux5/1
  odd_addr_w/1 -> Delay6/1
  Mux4/1 -> Dual Port RAM 1/4
  in_tvalid/1 -> addr_control/2, even_addr_w/2, odd_addr_w/2, Delay8/1, addr_r/2
  Mux2/1 -> Dual Port RAM 0/4
  Delay1/1 -> Dual Port RAM 0/2, Dual Port RAM 1/2
  Dual Port RAM 0/1 -> BitBasher/1
  Delay6/1 -> Mux2/3, Mux4/3
